simulink model "CCModel_62"  (R2024a)
settings: Solver=ode3  StartTime=0.0  StopTime=100  FixedStep=0.001  RelTol=1e-3  EnableMultiTasking=on
undefined symbols (not defined in the file or in its folder): DiscIntNeverNeededParam, Hecate_desVel1, Hecate_desVel2, Hecate_desVel3, Hecate_horShift, Hecate_period, Hecate_slope, Hecate_Transition1, Hecate_Transition2, Hecate_verShift, i, PME_qb, qb_map, RPM_qb, V
libraries: simulink x46
(part 11 of 11)

== system CCModel_62/Cruise Control/Version 6.1/Switches/Sigmoid_brake ==
  Change_time : Inport
  Old brake : Inport  Port=2
  New brake : Inport  Port=3
  Add : Sum
  Add1 : Sum
  Add2 : Sum
  Clock : Clock
  Constant : Constant
  Constant1 : Constant
  Constant2 : Constant
  Divide : Product  Inputs=/*
  Divide1 : Product  Inputs=**
  Divide2 : Product  Inputs=/*
  Divide3 : Product  Inputs=**
  Gain : Gain  Gain=1000
  Gain1 : Gain  Gain=0.001
  K : Constant
  Power{,1..3} (4 alike) : Math  Operator=pow
  Reciprocal : Product  Inputs=/
  Reciprocal1 : Product  Inputs=/
  Round : Rounding  Operator=round
  Scope : Scope  NumInputPorts=3
  Subtract : Sum  Inputs=-+
  Sum : Sum  Inputs=|-+
  brake_out : Outport
  wires:
  Power1/1 -> Scope/3, Add/1
  Add/1 -> Power/1
  Clock/1 -> Sum/2
  Constant/1 -> Add/2
  Sum/1 -> Gain/1  "Elapsed Time"
  Reciprocal/1 -> Power/2
  Power/1 -> Divide/1
  Divide/1 -> Divide1/1  "Sigmoid Function"
  Add1/1 -> Power2/1
  Power3/1 -> Add1/1
  K/1 -> Scope/2, Reciprocal/1, Power1/2, Reciprocal1/1, Power3/2
  Reciprocal1/1 -> Power2/2
  Power2/1 -> Divide2/1
  Constant1/1 -> Add1/2
  Change_time/1 -> Sum/1
  Constant2/1 -> Subtract/2
  Divide2/1 -> Subtract/1  "Sigmoid Function"
  Divide1/1 -> Add2/1
  Add2/1 -> brake_out/1
  New brake/1 -> Divide1/2
  Old brake/1 -> Divide3/2
  Subtract/1 -> Divide3/1
  Divide3/1 -> Add2/2
  Gain1/1 -> Power1/1, Divide/2, Scope/1, Divide2/2, Power3/1
  Gain/1 -> Round/1
  Round/1 -> Gain1/1

== system CCModel_62/Cruise Control/Version 6.1/Switches/Sigmoid_throttle ==
  Change_time : Inport
  Old thr : Inport  Port=2
  New thr : Inport  Port=3
  Add : Sum
  Add1 : Sum
  Add2 : Sum
  Clock : Clock
  Constant : Constant
  Constant1 : Constant
  Constant2 : Constant
  Divide : Product  Inputs=/*
  Divide1 : Product  Inputs=**
  Divide2 : Product  Inputs=/*
  Divide3 : Product  Inputs=**
  Gain : Gain  Gain=1000
  Gain1 : Gain  Gain=0.001
  K : Constant  Value=1.5
  Power{,1..3} (4 alike) : Math  Operator=pow
  Reciprocal : Product  Inputs=/
  Reciprocal1 : Product  Inputs=/
  Round : Rounding  Operator=round
  Scope : Scope  NumInputPorts=3
  Subtract : Sum  Inputs=-+
  Sum : Sum  Inputs=|-+
  throttle_out : Outport
  wires:
  Power1/1 -> Scope/3, Add/1
  Add/1 -> Power/1
  Clock/1 -> Sum/2
  Constant/1 -> Add/2
  Sum/1 -> Gain/1  "Elapsed Time"
  Reciprocal/1 -> Power/2
  Power/1 -> Divide/1
  Divide/1 -> Divide1/1  "Sigmoid Function"
  Add1/1 -> Power2/1
  Power3/1 -> Add1/1
  K/1 -> Scope/2, Reciprocal/1, Power1/2, Reciprocal1/1, Power3/2
  Reciprocal1/1 -> Power2/2
  Power2/1 -> Divide2/1
  Constant1/1 -> Add1/2
  Change_time/1 -> Sum/1
  Constant2/1 -> Subtract/2
  Divide2/1 -> Subtract/1  "Sigmoid Function"
  Divide1/1 -> Add2/1
  Add2/1 -> throttle_out/1
  New thr/1 -> Divide1/2
  Old thr/1 -> Divide3/2
  Subtract/1 -> Divide3/1
  Divide3/1 -> Add2/2
  Gain1/1 -> Power1/1, Divide/2, Scope/1, Divide2/2, Power3/1
  Gain/1 -> Round/1
  Round/1 -> Gain1/1

== system CCModel_62/Cruise Control/Version 6.2/Switches/Sigmoid_brake ==
  Change_time : Inport
  Old brake : Inport  Port=2
  New brake : Inport  Port=3
  Add : Sum
  Add1 : Sum
  Add2 : Sum
  Clock : Clock
  Constant : Constant
  Constant1 : Constant
  Constant2 : Constant
  Divide : Product  Inputs=/*
  Divide1 : Product  Inputs=**
  Divide2 : Product  Inputs=/*
  Divide3 : Product  Inputs=**
  Gain : Gain  Gain=1000
  Gain1 : Gain  Gain=0.001
  K : Constant  Value=1.5
  Power{,1..3} (4 alike) : Math  Operator=pow
  Reciprocal : Product  Inputs=/
  Reciprocal1 : Product  Inputs=/
  Round : Rounding  Operator=round
  Scope : Scope  NumInputPorts=3
  Subtract : Sum  Inputs=-+
  Sum : Sum  Inputs=|-+
  brake_out : Outport
  wires:
  Power1/1 -> Scope/3, Add/1
  Add/1 -> Power/1
  Clock/1 -> Sum/2
  Constant/1 -> Add/2
  Sum/1 -> Gain/1  "Elapsed Time"
  Reciprocal/1 -> Power/2
  Power/1 -> Divide/1
  Divide/1 -> Divide1/1  "Sigmoid Function"
  Add1/1 -> Power2/1
  Power3/1 -> Add1/1
  K/1 -> Scope/2, Reciprocal/1, Power1/2, Reciprocal1/1, Power3/2
  Reciprocal1/1 -> Power2/2
  Power2/1 -> Divide2/1
  Constant1/1 -> Add1/2
  Change_time/1 -> Sum/1
  Constant2/1 -> Subtract/2
  Divide2/1 -> Subtract/1  "Sigmoid Function"
  Divide1/1 -> Add2/1
  Add2/1 -> brake_out/1
  New brake/1 -> Divide1/2
  Old brake/1 -> Divide3/2
  Subtract/1 -> Divide3/1
  Divide3/1 -> Add2/2
  Gain1/1 -> Power1/1, Divide/2, Scope/1, Divide2/2, Power3/1
  Gain/1 -> Round/1
  Round/1 -> Gain1/1

== system CCModel_62/Cruise Control/Version 6.2/Switches/Sigmoid_throttle ==
  Change_time : Inport
  Old thr : Inport  Port=2
  New thr : Inport  Port=3
  Add : Sum
  Add1 : Sum
  Add2 : Sum
  Clock : Clock
  Constant : Constant
  Constant1 : Constant
  Constant2 : Constant
  Divide : Product  Inputs=/*
  Divide1 : Product  Inputs=**
  Divide2 : Product  Inputs=/*
  Divide3 : Product  Inputs=**
  Gain : Gain  Gain=1000
  Gain1 : Gain  Gain=0.001
  K : Constant  Value=1.5
  Power{,1..3} (4 alike) : Math  Operator=pow
  Reciprocal : Product  Inputs=/
  Reciprocal1 : Product  Inputs=/
  Round : Rounding  Operator=round
  Scope : Scope  NumInputPorts=3
  Subtract : Sum  Inputs=-+
  Sum : Sum  Inputs=|-+
  throttle_out : Outport
  wires:
  Power1/1 -> Scope/3, Add/1
  Add/1 -> Power/1
  Clock/1 -> Sum/2
  Constant/1 -> Add/2
  Sum/1 -> Gain/1  "Elapsed Time"
  Reciprocal/1 -> Power/2
  Power/1 -> Divide/1
  Divide/1 -> Divide1/1  "Sigmoid Function"
  Add1/1 -> Power2/1
  Power3/1 -> Add1/1
  K/1 -> Scope/2, Reciprocal/1, Power1/2, Reciprocal1/1, Power3/2
  Reciprocal1/1 -> Power2/2
  Power2/1 -> Divide2/1
  Constant1/1 -> Add1/2
  Change_time/1 -> Sum/1
  Constant2/1 -> Subtract/2
  Divide2/1 -> Subtract/1  "Sigmoid Function"
  Divide1/1 -> Add2/1
  Add2/1 -> throttle_out/1
  New thr/1 -> Divide1/2
  Old thr/1 -> Divide3/2
  Subtract/1 -> Divide3/1
  Divide3/1 -> Add2/2
  Gain1/1 -> Power1/1, Divide/2, Scope/1, Divide2/2, Power3/1
  Gain/1 -> Round/1
  Round/1 -> Gain1/1

== system CCModel_62/Cruise Control/Version 7.3/Detect Change/Change_Desired_Speed ==

== system CCModel_62/Cruise Control/Version 7.3/Detect Change/Driver Control ==

== system CCModel_62/Cruise Control/Version 7.3/Detect Change/Error_Equal_Zero ==

== system CCModel_62/Cruise Control/Version 7.3/PID Controller/Throttle Adjustment ==

== system CCModel_62/Powertrain/EM0/efficiency/divider ==
  In1 : Inport
  In2 : Inport  Port=2
  Fcn : Fcn  Expr="u(1) /  (u(2)+(u(2)==0) ) *(u(2)!=0)"
  Mux : Mux  Inputs=2
  Out1 : Outport
  wires:
  In2/1 -> Mux/2
  Fcn/1 -> Out1/1
  In1/1 -> Mux/1
  Mux/1 -> Fcn/1

== system CCModel_62/Powertrain/EM0/efficiency/divider1 ==
  In1 : Inport
  In2 : Inport  Port=2
  Fcn : Fcn  Expr="u(1) /  (u(2)+(u(2)==0) ) *(u(2)!=0)"
  Mux : Mux  Inputs=2
  Out1 : Outport
  wires:
  In2/1 -> Mux/2
  Fcn/1 -> Out1/1
  In1/1 -> Mux/1
  Mux/1 -> Fcn/1

== system CCModel_62/Powertrain/EM1/efficiency/divider ==
  In1 : Inport
  In2 : Inport  Port=2
  Fcn : Fcn  Expr="u(1) /  (u(2)+(u(2)==0) ) *(u(2)!=0)"
  Mux : Mux  Inputs=2
  Out1 : Outport
  wires:
  In2/1 -> Mux/2
  Fcn/1 -> Out1/1
  In1/1 -> Mux/1
  Mux/1 -> Fcn/1

== system CCModel_62/Powertrain/EM1/efficiency/divider1 ==
  In1 : Inport
  In2 : Inport  Port=2
  Fcn : Fcn  Expr="u(1) /  (u(2)+(u(2)==0) ) *(u(2)!=0)"
  Mux : Mux  Inputs=2
  Out1 : Outport
  wires:
  In2/1 -> Mux/2
  Fcn/1 -> Out1/1
  In1/1 -> Mux/1
  Mux/1 -> Fcn/1

== system CCModel_62/Powertrain/EM2/efficiency/divider ==
  In1 : Inport
  In2 : Inport  Port=2
  Fcn : Fcn  Expr="u(1) /  (u(2)+(u(2)==0) ) *(u(2)!=0)"
  Mux : Mux  Inputs=2
  Out1 : Outport
  wires:
  In2/1 -> Mux/2
  Fcn/1 -> Out1/1
  In1/1 -> Mux/1
  Mux/1 -> Fcn/1

== system CCModel_62/Powertrain/EM2/efficiency/divider1 ==
  In1 : Inport
  In2 : Inport  Port=2
  Fcn : Fcn  Expr="u(1) /  (u(2)+(u(2)==0) ) *(u(2)!=0)"
  Mux : Mux  Inputs=2
  Out1 : Outport
  wires:
  In2/1 -> Mux/2
  Fcn/1 -> Out1/1
  In1/1 -> Mux/1
  Mux/1 -> Fcn/1

== system CCModel_62/Powertrain/EM3/efficiency/divider ==
  In1 : Inport
  In2 : Inport  Port=2
  Fcn : Fcn  Expr="u(1) /  (u(2)+(u(2)==0) ) *(u(2)!=0)"
  Mux : Mux  Inputs=2
  Out1 : Outport
  wires:
  In2/1 -> Mux/2
  Fcn/1 -> Out1/1
  In1/1 -> Mux/1
  Mux/1 -> Fcn/1

== system CCModel_62/Powertrain/EM3/efficiency/divider1 ==
  In1 : Inport
  In2 : Inport  Port=2
  Fcn : Fcn  Expr="u(1) /  (u(2)+(u(2)==0) ) *(u(2)!=0)"
  Mux : Mux  Inputs=2
  Out1 : Outport
  wires:
  In2/1 -> Mux/2
  Fcn/1 -> Out1/1
  In1/1 -> Mux/1
  Mux/1 -> Fcn/1

== system CCModel_62/Powertrain/EM4Front/efficiency/divider ==
  In1 : Inport
  In2 : Inport  Port=2
  Fcn : Fcn  Expr="u(1) /  (u(2)+(u(2)==0) ) *(u(2)!=0)"
  Mux : Mux  Inputs=2
  Out1 : Outport
  wires:
  In2/1 -> Mux/2
  Fcn/1 -> Out1/1
  In1/1 -> Mux/1
  Mux/1 -> Fcn/1

== system CCModel_62/Powertrain/EM4Front/efficiency/divider1 ==
  In1 : Inport
  In2 : Inport  Port=2
  Fcn : Fcn  Expr="u(1) /  (u(2)+(u(2)==0) ) *(u(2)!=0)"
  Mux : Mux  Inputs=2
  Out1 : Outport
  wires:
  In2/1 -> Mux/2
  Fcn/1 -> Out1/1
  In1/1 -> Mux/1
  Mux/1 -> Fcn/1

== system CCModel_62/Powertrain/EM4Rear/efficiency/divider ==
  In1 : Inport
  In2 : Inport  Port=2
  Fcn : Fcn  Expr="u(1) /  (u(2)+(u(2)==0) ) *(u(2)!=0)"
  Mux : Mux  Inputs=2
  Out1 : Outport
  wires:
  In2/1 -> Mux/2
  Fcn/1 -> Out1/1
  In1/1 -> Mux/1
  Mux/1 -> Fcn/1

== system CCModel_62/Powertrain/EM4Rear/efficiency/divider1 ==
  In1 : Inport
  In2 : Inport  Port=2
  Fcn : Fcn  Expr="u(1) /  (u(2)+(u(2)==0) ) *(u(2)!=0)"
  Mux : Mux  Inputs=2
  Out1 : Outport
  wires:
  In2/1 -> Mux/2
  Fcn/1 -> Out1/1
  In1/1 -> Mux/1
  Mux/1 -> Fcn/1

== system CCModel_62/Powertrain/EMR/efficiency/divider ==
  In1 : Inport
  In2 : Inport  Port=2
  Fcn : Fcn  Expr="u(1) /  (u(2)+(u(2)==0) ) *(u(2)!=0)"
  Mux : Mux  Inputs=2
  Out1 : Outport
  wires:
  In2/1 -> Mux/2
  Fcn/1 -> Out1/1
  In1/1 -> Mux/1
  Mux/1 -> Fcn/1

== system CCModel_62/Powertrain/EMR/efficiency/divider1 ==
  In1 : Inport
  In2 : Inport  Port=2
  Fcn : Fcn  Expr="u(1) /  (u(2)+(u(2)==0) ) *(u(2)!=0)"
  Mux : Mux  Inputs=2
  Out1 : Outport
  wires:
  In2/1 -> Mux/2
  Fcn/1 -> Out1/1
  In1/1 -> Mux/1
  Mux/1 -> Fcn/1

== system CCModel_62/Powertrain/EMS/efficiency/divider ==
  In1 : Inport
  In2 : Inport  Port=2
  Fcn : Fcn  Expr="u(1) /  (u(2)+(u(2)==0) ) *(u(2)!=0)"
  Mux : Mux  Inputs=2
  Out1 : Outport
  wires:
  In2/1 -> Mux/2
  Fcn/1 -> Out1/1
  In1/1 -> Mux/1
  Mux/1 -> Fcn/1

== system CCModel_62/Powertrain/EMS/efficiency/divider1 ==
  In1 : Inport
  In2 : Inport  Port=2
  Fcn : Fcn  Expr="u(1) /  (u(2)+(u(2)==0) ) *(u(2)!=0)"
  Mux : Mux  Inputs=2
  Out1 : Outport
  wires:
  In2/1 -> Mux/2
  Fcn/1 -> Out1/1
  In1/1 -> Mux/1
  Mux/1 -> Fcn/1

== system CCModel_62/Powertrain/EV/Motor Efficiency/  ==
  In1 : Inport
  In2 : Inport  Port=2
  Fcn : Fcn  Expr=u[1]/(u[2]+(u[2]==0))*(u[2]!=0)
  Mux : Mux  Inputs=2
  Out1 : Outport  VectorParamsAs1DForOutWhenUnconnected=off
  wires:
  In1/1 -> Mux/1
  In2/1 -> Mux/2
  Mux/1 -> Fcn/1
  Fcn/1 -> Out1/1

== system CCModel_62/Powertrain/GEN/efficiency/divider ==
  In1 : Inport
  In2 : Inport  Port=2
  Fcn : Fcn  Expr="u(1) /  (u(2)+(u(2)==0) ) *(u(2)!=0)"
  Mux : Mux  Inputs=2
  Out1 : Outport
  wires:
  In2/1 -> Mux/2
  Fcn/1 -> Out1/1
  In1/1 -> Mux/1
  Mux/1 -> Fcn/1

== system CCModel_62/Powertrain/GEN/efficiency/divider1 ==
  In1 : Inport
  In2 : Inport  Port=2
  Fcn : Fcn  Expr="u(1) /  (u(2)+(u(2)==0) ) *(u(2)!=0)"
  Mux : Mux  Inputs=2
  Out1 : Outport
  wires:
  In2/1 -> Mux/2
  Fcn/1 -> Out1/1
  In1/1 -> Mux/1
  Mux/1 -> Fcn/1

== system CCModel_62/Powertrain/MOT/efficiency/divider ==
  In1 : Inport
  In2 : Inport  Port=2
  Fcn : Fcn  Expr="u(1) /  (u(2)+(u(2)==0) ) *(u(2)!=0)"
  Mux : Mux  Inputs=2
  Out1 : Outport
  wires:
  In2/1 -> Mux/2
  Fcn/1 -> Out1/1
  In1/1 -> Mux/1
  Mux/1 -> Fcn/1

== system CCModel_62/Powertrain/MOT/efficiency/divider1 ==
  In1 : Inport
  In2 : Inport  Port=2
  Fcn : Fcn  Expr="u(1) /  (u(2)+(u(2)==0) ) *(u(2)!=0)"
  Mux : Mux  Inputs=2
  Out1 : Outport
  wires:
  In2/1 -> Mux/2
  Fcn/1 -> Out1/1
  In1/1 -> Mux/1
  Mux/1 -> Fcn/1

== stateflow chart CCModel_62/Requirements Table ==
  (default) -> (junction 1073742629)
  (junction 1073742629) -> (junction 1073742630) : {
      | % SF_REQ_REV_07
      | }
  (junction 1073742630) -> (junction 1073742632) : {
      | % ExcEvals:
      | % PriEvals:
      | }
  (junction 1073742632) -> (junction 1073742634) : {
      | % HEADER_ASSIGNMENTS
      |
      | }
  (junction 1073742634) -> (junction 1073742636) : {
      | % START_A_4
      | }
  (junction 1073742636) -> (junction 1073742638) : {
      | }
  (junction 1073742638) -> (junction 1073742640)
  (junction 1073742640) -> (junction 1073742642) : {
      | }
  (junction 1073742642) -> (junction 1073742644) : {
      | % END_A_4
      | }
  (junction 1073742644) -> (junction 1073742646) : {
      | % START_R_1
      | }
  (junction 1073742646) -> (junction 1073742648) : {
      | }
  (junction 1073742648) -> (junction 1073742650)
  (junction 1073742650) -> (junction 1073742652) [order 1] : [duration((((throttle) < (1))) && (((brake) < (1)))) >= 0.5]
  (junction 1073742650) -> (junction 1073742658) [order 2]
  (junction 1073742652) -> (junction 1073742654) : {
      | reqtable_postcondition((((long_acc) >= (-3.5) && (long_acc) <= (5))), 'R:1');
      |
      |
      | }
  (junction 1073742654) -> (junction 1073742656) : {
      | }
  (junction 1073742656) -> (junction 1073742658)
  (junction 1073742658) -> (junction 1073742660)
  (junction 1073742660) -> (junction 1073742662) : {
      | % END_R_1
      | }
  (junction 1073742662) -> (junction 1073742664) : {
      | % START_R_7
      | }
  (junction 1073742664) -> (junction 1073742666) : {
      | }
  (junction 1073742666) -> (junction 1073742668)
  (junction 1073742668) -> (junction 1073742670) [order 1] : [duration((((throttle) < (1))) && (((brake) < (1)))) >= 0.5]
  (junction 1073742668) -> (junction 1073742676) [order 2]
  (junction 1073742670) -> (junction 1073742672) : {
      | reqtable_postcondition((abs((jerk)) <10 ), 'R:2');
      |
      |
      | }
  (junction 1073742672) -> (junction 1073742674) : {
      | }
  (junction 1073742674) -> (junction 1073742676)
  (junction 1073742676) -> (junction 1073742678)
  (junction 1073742678) -> (junction 1073742680) : {
      | % END_R_7
      | }
  (junction 1073742680) -> (junction 1073742682) : {
      | % START_R_10
      | }
  (junction 1073742682) -> (junction 1073742684) : {
      | }
  (junction 1073742684) -> (junction 1073742686)
  (junction 1073742686) -> (junction 1073742688) [order 1] : [duration((((throttle) < (1))) && (((brake) < (1)))) >= 0.5]
  (junction 1073742686) -> (junction 1073742694) [order 2]
  (junction 1073742688) -> (junction 1073742690) : {
      | reqtable_postcondition((abs((pitch_acc)) <3), 'R:3');
      |
      |
      | }
  (junction 1073742690) -> (junction 1073742692) : {
      | }
  (junction 1073742692) -> (junction 1073742694)
  (junction 1073742694) -> (junction 1073742696)
  (junction 1073742696) -> (junction 1073742698) : {
      | % END_R_10
      | }
  (junction 1073742698) -> (junction 1073742700) : {
      | % START_R_13
      | }
  (junction 1073742700) -> (junction 1073742702) : {
      | }
  (junction 1073742702) -> (junction 1073742704)
  (junction 1073742704) -> (junction 1073742706) [order 1] : [duration((((throttle) < (1))) && (((brake) < (1))) && (~changeTrigger)) >= 30]
  (junction 1073742704) -> (junction 1073742712) [order 2]
  (junction 1073742706) -> (junction 1073742708) : {
      | reqtable_postcondition((abs(des_vel - long_vel) < 3), 'R:4');
      |
      |
      | }
  (junction 1073742708) -> (junction 1073742710) : {
      | }
  (junction 1073742710) -> (junction 1073742712)
  (junction 1073742712) -> (junction 1073742714)
  (junction 1073742714) -> (junction 1073742716) : {
      | % END_R_13
      | }
  (junction 1073742716) -> (junction 1073742718) : {
      | % START_R_16
      | }
  (junction 1073742718) -> (junction 1073742720) : {
      | }
  (junction 1073742720) -> (junction 1073742722)
  (junction 1073742722) -> (junction 1073742724) [order 1] : [(((throttle) < (100000000))) && (((brake) < (100000000)))]
  (junction 1073742722) -> (junction 1073742730) [order 2]
  (junction 1073742724) -> (junction 1073742726) : {
      | reqtable_postcondition((((long_acc) < (100000000))) && (((jerk) < (100000000))) && (((pitch_acc) < (100000000))) && (des_vel < 100000000 && long_vel < 100000000 ), 'R:5');
      |
      |
      | }
  (junction 1073742726) -> (junction 1073742728) : {
      | }
  (junction 1073742728) -> (junction 1073742730)
  (junction 1073742730) -> (junction 1073742732)
  (junction 1073742732) -> (junction 1073742734) : {
      | % END_R_16
      | }
  data: brake input; throttle input; long_acc input; jerk input; des_vel input; long_vel input; pitch_acc input; changeTrigger input

== stateflow chart CCModel_62/Test Sequence1 ==
  state TS1
    state step_1
      throttle_const = 0;
      brake_const=0;
      desired_velocity = Hecate_desVel1;
      grade = 0;
    state step_2
      desired_velocity = Hecate_desVel2;
    (default) -> TS1.step_1
    TS1.step_1 -> TS1.step_2 : [
        | et >= Hecate_Transition1
        | ]
  state TS2
    state step_1
      throttle_const = 100;
      brake_const = 0;
      desired_velocity = Hecate_desVel1;
      grade = 0;
    state step_2
      throttle_const = 70 - 0.1*et(msec);
    state step_3
      %do nothing
    state step_4
      desired_velocity = Hecate_desVel2;
    (default) -> TS2.step_1
    TS2.step_1 -> TS2.step_2 : [
        | velocity >= 50
        | ]
    TS2.step_2 -> TS2.step_3 : [
        | throttle_const <= 0
        | ]
    TS2.step_3 -> TS2.step_4 : [
        | et>=Hecate_Transition1
        | ]
  state TS3
    state step_1
      steer_angle = 0;
      throttle_const = 100;
      brake_const = 0;
      desired_velocity = Hecate_desVel1;
      grade = 0;
    state step_2
      throttle_const = 70 - 0.1*et(msec);
    state step_3
      %do nothing
    state step_4
      desired_velocity = Hecate_desVel2;
    state step_5
      desired_velocity = Hecate_desVel3;
    (default) -> TS3.step_1
    TS3.step_1 -> TS3.step_2 : [
        | velocity >= 50
        | ]
    TS3.step_2 -> TS3.step_3 : [
        | throttle_const <= 0
        | ]
    TS3.step_3 -> TS3.step_4 : [
        | et>=Hecate_Transition1
        | ]
    TS3.step_4 -> TS3.step_5 : [
        | et>=Hecate_Transition2
        | ]
  state TS4
    state step_1
      throttle_const = 100;
      brake_const = 0;
      desired_velocity = Hecate_desVel1;
      grade = Hecate_slope;
    state step_2
      throttle_const = 70 - 0.1*et(msec);
    state step_3
      %do nothing
    state step_4
      desired_velocity = Hecate_desVel2;
    (default) -> TS4.step_1
    TS4.step_1 -> TS4.step_2 : [
        | velocity >= 50
        | ]
    TS4.step_2 -> TS4.step_3 : [
        | throttle_const <= 0
        | ]
    TS4.step_3 -> TS4.step_4 : [
        | et>=Hecate_Transition1
        | ]
  state TS5
    state step_1
      steer_angle = 0;
      throttle_const = 100;
      brake_const = 0;
      desired_velocity = Hecate_desVel1;
      grade = Hecate_slope;
    state step_2
      throttle_const = 70 - 0.1*et(msec);
    state step_3
      %do nothing
    state step_4
      desired_velocity = Hecate_desVel2;
    state step_5
      desired_velocity = Hecate_desVel3;
    (default) -> TS5.step_1
    TS5.step_1 -> TS5.step_2 : [
        | velocity >= 50
        | ]
    TS5.step_2 -> TS5.step_3 : [
        | throttle_const <= 0
        | ]
    TS5.step_3 -> TS5.step_4 : [
        | et>=Hecate_Transition1
        | ]
    TS5.step_4 -> TS5.step_5 : [
        | et>=Hecate_Transition2
        | ]
  state TS6
    state Start_Up
      steer_angle = 0;
      throttle_const = 100;
      brake_const = 0;
      desired_velocity = Hecate_desVel1;
      grade = Hecate_slope*sin(pi*t/Hecate_period + Hecate_horShift) + Hecate_verShift;
    state Release_Throttle
      throttle_const = 70 - 0.1*et(msec);
      grade = Hecate_slope*sin(pi*t/Hecate_period + Hecate_horShift) + Hecate_verShift;
    state Initial_Step
      desired_velocity = Hecate_desVel1;
      grade = Hecate_slope*sin(pi*t/Hecate_period + Hecate_horShift) + Hecate_verShift;
    state Intermediary_Step
      desired_velocity = Hecate_desVel2;
      grade = Hecate_slope*sin(pi*t/Hecate_period + Hecate_horShift) + Hecate_verShift;
    state Final_Step
      desired_velocity = Hecate_desVel3;
      grade = Hecate_slope*sin(pi*t/Hecate_period + Hecate_horShift) + Hecate_verShift;
    (default) -> Start_Up
    Start_Up -> Release_Throttle : [
        | velocity >= 50
        | ]
    Release_Throttle -> Initial_Step : [
        | throttle_const <= 0
        | ]
    Initial_Step -> Intermediary_Step : [
        | et>=Hecate_Transition1
        | ]
    Intermediary_Step -> Final_Step : [
        | et>=Hecate_Transition2
        | ]
  state Scenario_1
    state step_1
    state step_2
    (default) -> Scenario_1.step_1
    Scenario_1.step_1 -> Scenario_1.step_2
  (default) -> TS1 [order 1] : [Active_Scenario_Index == 1]
  (default) -> TS2 [order 2] : [Active_Scenario_Index == 2]
  (default) -> TS3 [order 3] : [Active_Scenario_Index == 3]
  (default) -> TS4 [order 4] : [Active_Scenario_Index == 4]
  (default) -> TS5 [order 5] : [Active_Scenario_Index == 5]
  (default) -> TS6 [order 6] : [Active_Scenario_Index == 6]
  (default) -> Scenario_1 [order 7] : {assert(Active_Scenario_Index == 7,'The value of Scenario Parameter ''Active_Scenario_Index'' is not valid. Use the index of the scenario to specify it.')}
  data: steer_angle output; throttle_const output; brake_const output; Active_Scenario_Index parameter =4; Hecate_desVel2 parameter; Hecate_desVel1 parameter; desired_velocity output; Hecate_desVel3 parameter; Hecate_Transition1 parameter; Hecate_Transition2 parameter; velocity input; grade output; Hecate_slope parameter; Hecate_horShift parameter; Hecate_verShift parameter; Hecate_period parameter

== stateflow chart CCModel_62/FitnessConverter_Hecate ==
  state Requirement_1 [parallel]
    settings: executionOrder=1
    state Default
      rob1 = Inf;
    state Wait
      rob1 = Inf;
    state Verify
      rob1 = min( 5-(long_acc),(long_acc-( -3.5)));
    (default) -> (junction 14)
    (junction 14) -> Requirement_1.Wait [order 2]
    (junction 14) -> Requirement_1.Default [order 1] : [~((throttle<1) && (brake<1))]
    Requirement_1.Default -> Requirement_1.Wait : [(throttle<1) && (brake<1)]
    Requirement_1.Wait -> Requirement_1.Default [order 1] : [~((throttle<1) && (brake<1))]
    Requirement_1.Verify -> Requirement_1.Default : [~((throttle<1) && (brake<1))]
    Requirement_1.Wait -> Requirement_1.Verify [order 2] : [et >= 0.5]
  state Requirement_2 [parallel]
    settings: executionOrder=2
    state Default
      rob2 = Inf;
    state Wait
      rob2 = Inf;
    state Verify
      rob2 = 10-((abs(jerk)));
    (default) -> (junction 26)
    (junction 26) -> Requirement_2.Wait [order 2]
    (junction 26) -> Requirement_2.Default [order 1] : [~((throttle<1) && (brake<1))]
    Requirement_2.Default -> Requirement_2.Wait : [(throttle<1) && (brake<1)]
    Requirement_2.Wait -> Requirement_2.Default [order 1] : [~((throttle<1) && (brake<1))]
    Requirement_2.Verify -> Requirement_2.Default : [~((throttle<1) && (brake<1))]
    Requirement_2.Wait -> Requirement_2.Verify [order 2] : [et >= 0.5]
  state Requirement_3 [parallel]
    settings: executionOrder=3
    state Default
      rob3 = Inf;
    state Wait
      rob3 = Inf;
    state Verify
      rob3 = 3-((abs(pitch_acc)));
    (default) -> (junction 38)
    (junction 38) -> Requirement_3.Wait [order 2]
    (junction 38) -> Requirement_3.Default [order 1] : [~((throttle<1) && (brake<1))]
    Requirement_3.Default -> Requirement_3.Wait : [(throttle<1) && (brake<1)]
    Requirement_3.Wait -> Requirement_3.Default [order 1] : [~((throttle<1) && (brake<1))]
    Requirement_3.Verify -> Requirement_3.Default : [~((throttle<1) && (brake<1))]
    Requirement_3.Wait -> Requirement_3.Verify [order 2] : [et >= 0.5]
  state Requirement_4 [parallel]
    settings: executionOrder=4
    state Default
      rob4 = Inf;
    state Wait
      rob4 = Inf;
    state Verify
      rob4 = 3-((abs(des_vel-long_vel)));
    (default) -> (junction 50)
    (junction 50) -> Requirement_4.Wait [order 2]
    (junction 50) -> Requirement_4.Default [order 1] : [~((throttle<1) && (brake<1) && (~changeTrigger))]
    Requirement_4.Default -> Requirement_4.Wait : [(throttle<1) && (brake<1) && (~changeTrigger)]
    Requirement_4.Wait -> Requirement_4.Default [order 1] : [~((throttle<1) && (brake<1) && (~changeTrigger))]
    Requirement_4.Verify -> Requirement_4.Default : [~((throttle<1) && (brake<1) && (~changeTrigger))]
    Requirement_4.Wait -> Requirement_4.Verify [order 2] : [et >= 30]
  data: brake input; throttle input; long_acc input; jerk input; des_vel input; long_vel input; pitch_acc input; changeTrigger input; rob1 output double =Inf; rob2 output double =Inf; rob3 output double =Inf; rob4 output double =Inf

== stateflow chart CCModel_62/Test Assessment1 ==
  state Func
    state Driver_Active
      %Do nothing
      settings: description=Recent brake
    state Buffer
      %Wait
    state CC_Active
      %Nothing
      settings: description=Start
      state Wait_Period
        %Nothing
        settings: description=Recent change (start)
      state Time_Threshold
        verify(abs(desired_velocity-long_vel_lp) <= 3)
        settings: description=No recent change
      state Refresh
        %Nothing
      Func.CC_Active.Refresh -> (junction 350) : [
          | et >= 0.5
          | ]
      (default) -> Func.CC_Active.Wait_Period
      Func.CC_Active.Wait_Period -> (junction 344) [order 2] : [
          | hasChanged(desired_velocity)
          | ]
      (junction 348) -> Func.CC_Active.Wait_Period
      (junction 344) -> (junction 342)
      Func.CC_Active.Wait_Period -> Func.CC_Active.Time_Threshold [order 1] : [
          | et >= 29.5
          | ]
      Func.CC_Active.Time_Threshold -> Func.CC_Active.Refresh : [
          | hasChanged(desired_velocity)
          | ]
      (junction 342) -> Func.CC_Active.Refresh
      (junction 350) -> (junction 348)
    Func.CC_Active -> (junction 338) : [
        | brake >= 1 || throttle >= 1
        | ]
    (default) -> Func.Driver_Active
    (junction 336) -> Func.Driver_Active
    Func.Driver_Active -> Func.Buffer : [
        | brake < 1 && throttle < 1
        | ]
    Func.Buffer -> Func.CC_Active : [
        | et >= 0.5
        | ]
    (junction 338) -> (junction 336)
  state DrivAndFunc
    state Driver_Active
      %Do nothing
      settings: description=Recent brake
    state Buffer
      %Wait
    state CC_Active
      verify(long_acc_lp <= 5)
      verify(long_acc_lp >= -3.5)
      verify(abs(pitch_acc_lp) <=3)
      verify(abs(long_jerk) <= 10)
      settings: description=Start
      state Wait_Period
        %Nothing
        settings: description=Recent change (start)
      state Time_Threshold
        verify(abs(desired_velocity-long_vel_lp) <= 3)
        settings: description=No recent change
      state Refresh
        %Nothing
      DrivAndFunc.CC_Active.Refresh -> (junction 260) : [
          | et >= 0.5
          | ]
      (default) -> DrivAndFunc.CC_Active.Wait_Period
      DrivAndFunc.CC_Active.Wait_Period -> (junction 254) [order 2] : [
          | hasChanged(desired_velocity)
          | ]
      (junction 258) -> DrivAndFunc.CC_Active.Wait_Period
      (junction 254) -> (junction 252)
      DrivAndFunc.CC_Active.Wait_Period -> DrivAndFunc.CC_Active.Time_Threshold [order 1] : [
          | et >= 29.5
          | ]
      DrivAndFunc.CC_Active.Time_Threshold -> DrivAndFunc.CC_Active.Refresh : [
          | hasChanged(desired_velocity)
          | ]
      (junction 252) -> DrivAndFunc.CC_Active.Refresh
      (junction 260) -> (junction 258)
    DrivAndFunc.CC_Active -> (junction 248) : [
        | brake >= 1 || throttle >= 1
        | ]
    (default) -> DrivAndFunc.Driver_Active
    (junction 246) -> DrivAndFunc.Driver_Active
    DrivAndFunc.Driver_Active -> DrivAndFunc.Buffer : [
        | brake < 1 && throttle < 1
        | ]
    DrivAndFunc.Buffer -> DrivAndFunc.CC_Active : [
        | et >= 0.5
        | ]
    (junction 248) -> (junction 246)
  (default) -> Func [order 1] : [Active_Scenario_Index == 1]
  (default) -> DrivAndFunc [order 2] : {assert(Active_Scenario_Index == 2,'The value of Scenario Parameter ''Active_Scenario_Index'' is not valid. Use the index of the scenario to specify it.')}
  data: long_jerk input; long_acc_lp input; long_vel_lp input; pitch_acc_lp input; Active_Scenario_Index parameter =1; brake input; throttle input; desired_velocity input

== stateflow chart CCModel_62/Requirements Table1 ==
  (default) -> (junction 1073742629)
  (junction 1073742629) -> (junction 1073742630) : {
      | % SF_REQ_REV_07
      | }
  (junction 1073742630) -> (junction 1073742632) : {
      | % ExcEvals:
      | % PriEvals:
      | }
  (junction 1073742632) -> (junction 1073742634) : {
      | % HEADER_ASSIGNMENTS
      |
      | }
  (junction 1073742634) -> (junction 1073742636) : {
      | % START_A_4
      | }
  (junction 1073742636) -> (junction 1073742638) : {
      | }
  (junction 1073742638) -> (junction 1073742640)
  (junction 1073742640) -> (junction 1073742642) : {
      | }
  (junction 1073742642) -> (junction 1073742644) : {
      | % END_A_4
      | }
  (junction 1073742644) -> (junction 1073742646) : {
      | % START_R_1
      | }
  (junction 1073742646) -> (junction 1073742648) : {
      | }
  (junction 1073742648) -> (junction 1073742650)
  (junction 1073742650) -> (junction 1073742652) [order 1] : [duration((((throttle) < (1))) && (((brake) < (1)))) >= 0.7]
  (junction 1073742650) -> (junction 1073742658) [order 2]
  (junction 1073742652) -> (junction 1073742654) : {
      | reqtable_postcondition((((long_acc) >= (-3.5) && (long_acc) <= (5))), 'R:1');
      |
      |
      | }
  (junction 1073742654) -> (junction 1073742656) : {
      | }
  (junction 1073742656) -> (junction 1073742658)
  (junction 1073742658) -> (junction 1073742660)
  (junction 1073742660) -> (junction 1073742662) : {
      | % END_R_1
      | }
  (junction 1073742662) -> (junction 1073742664) : {
      | % START_R_7
      | }
  (junction 1073742664) -> (junction 1073742666) : {
      | }
  (junction 1073742666) -> (junction 1073742668)
  (junction 1073742668) -> (junction 1073742670) [order 1] : [duration((((throttle) < (1))) && (((brake) < (1)))) >= 0.7]
  (junction 1073742668) -> (junction 1073742676) [order 2]
  (junction 1073742670) -> (junction 1073742672) : {
      | reqtable_postcondition((abs((jerk)) <10 ), 'R:2');
      |
      |
      | }
  (junction 1073742672) -> (junction 1073742674) : {
      | }
  (junction 1073742674) -> (junction 1073742676)
  (junction 1073742676) -> (junction 1073742678)
  (junction 1073742678) -> (junction 1073742680) : {
      | % END_R_7
      | }
  (junction 1073742680) -> (junction 1073742682) : {
      | % START_R_10
      | }
  (junction 1073742682) -> (junction 1073742684) : {
      | }
  (junction 1073742684) -> (junction 1073742686)
  (junction 1073742686) -> (junction 1073742688) [order 1] : [duration((((throttle) < (1))) && (((brake) < (1)))) >= 0.7]
  (junction 1073742686) -> (junction 1073742694) [order 2]
  (junction 1073742688) -> (junction 1073742690) : {
      | reqtable_postcondition((abs((pitch_acc)) <3), 'R:3');
      |
      |
      | }
  (junction 1073742690) -> (junction 1073742692) : {
      | }
  (junction 1073742692) -> (junction 1073742694)
  (junction 1073742694) -> (junction 1073742696)
  (junction 1073742696) -> (junction 1073742698) : {
      | % END_R_10
      | }
  (junction 1073742698) -> (junction 1073742700) : {
      | % START_R_13
      | }
  (junction 1073742700) -> (junction 1073742702) : {
      | }
  (junction 1073742702) -> (junction 1073742704)
  (junction 1073742704) -> (junction 1073742706) [order 1] : [duration((((throttle) < (1))) && (((brake) < (1))) && (~changeTrigger)) >= 30]
  (junction 1073742704) -> (junction 1073742712) [order 2]
  (junction 1073742706) -> (junction 1073742708) : {
      | reqtable_postcondition((abs(des_vel - long_vel) < 3), 'R:4');
      |
      |
      | }
  (junction 1073742708) -> (junction 1073742710) : {
      | }
  (junction 1073742710) -> (junction 1073742712)
  (junction 1073742712) -> (junction 1073742714)
  (junction 1073742714) -> (junction 1073742716) : {
      | % END_R_13
      | }
  (junction 1073742716) -> (junction 1073742718) : {
      | % START_R_16
      | }
  (junction 1073742718) -> (junction 1073742720) : {
      | }
  (junction 1073742720) -> (junction 1073742722)
  (junction 1073742722) -> (junction 1073742724) [order 1] : [(((throttle) < (100000000))) && (((brake) < (100000000)))]
  (junction 1073742722) -> (junction 1073742730) [order 2]
  (junction 1073742724) -> (junction 1073742726) : {
      | reqtable_postcondition((((long_acc) < (100000000))) && (((jerk) < (100000000))) && (((pitch_acc) < (100000000))) && (des_vel < 100000000 && long_vel < 100000000 ), 'R:5');
      |
      |
      | }
  (junction 1073742726) -> (junction 1073742728) : {
      | }
  (junction 1073742728) -> (junction 1073742730)
  (junction 1073742730) -> (junction 1073742732)
  (junction 1073742732) -> (junction 1073742734) : {
      | % END_R_16
      | }
  data: brake input; throttle input; long_acc input; jerk input; des_vel input; long_vel input; pitch_acc input; changeTrigger input

== stateflow chart CCModel_62/Requirements Table2 ==
  (default) -> (junction 1073742629)
  (junction 1073742629) -> (junction 1073742630) : {
      | % SF_REQ_REV_07
      | }
  (junction 1073742630) -> (junction 1073742632) : {
      | % ExcEvals:
      | % PriEvals:
      | }
  (junction 1073742632) -> (junction 1073742634) : {
      | % HEADER_ASSIGNMENTS
      |
      | }
  (junction 1073742634) -> (junction 1073742636) : {
      | % START_A_4
      | }
  (junction 1073742636) -> (junction 1073742638) : {
      | }
  (junction 1073742638) -> (junction 1073742640)
  (junction 1073742640) -> (junction 1073742642) : {
      | }
  (junction 1073742642) -> (junction 1073742644) : {
      | % END_A_4
      | }
  (junction 1073742644) -> (junction 1073742646) : {
      | % START_R_1
      | }
  (junction 1073742646) -> (junction 1073742648) : {
      | }
  (junction 1073742648) -> (junction 1073742650)
  (junction 1073742650) -> (junction 1073742652) [order 1] : [duration((((throttle) < (1))) && (((brake) < (1)))) >= 0.7]
  (junction 1073742650) -> (junction 1073742658) [order 2]
  (junction 1073742652) -> (junction 1073742654) : {
      | reqtable_postcondition((((long_acc) >= (-3.5) && (long_acc) <= (5))), 'R:1');
      |
      |
      | }
  (junction 1073742654) -> (junction 1073742656) : {
      | }
  (junction 1073742656) -> (junction 1073742658)
  (junction 1073742658) -> (junction 1073742660)
  (junction 1073742660) -> (junction 1073742662) : {
      | % END_R_1
      | }
  (junction 1073742662) -> (junction 1073742664) : {
      | % START_R_7
      | }
  (junction 1073742664) -> (junction 1073742666) : {
      | }
  (junction 1073742666) -> (junction 1073742668)
  (junction 1073742668) -> (junction 1073742670) [order 1] : [duration((((throttle) < (1))) && (((brake) < (1)))) >= 0.7]
  (junction 1073742668) -> (junction 1073742676) [order 2]
  (junction 1073742670) -> (junction 1073742672) : {
      | reqtable_postcondition((abs((jerk)) <10 ), 'R:2');
      |
      |
      | }
  (junction 1073742672) -> (junction 1073742674) : {
      | }
  (junction 1073742674) -> (junction 1073742676)
  (junction 1073742676) -> (junction 1073742678)
  (junction 1073742678) -> (junction 1073742680) : {
      | % END_R_7
      | }
  (junction 1073742680) -> (junction 1073742682) : {
      | % START_R_10
      | }
  (junction 1073742682) -> (junction 1073742684) : {
      | }
  (junction 1073742684) -> (junction 1073742686)
  (junction 1073742686) -> (junction 1073742688) [order 1] : [duration((((throttle) < (1))) && (((brake) < (1)))) >= 0.7]
  (junction 1073742686) -> (junction 1073742694) [order 2]
  (junction 1073742688) -> (junction 1073742690) : {
      | reqtable_postcondition((abs((pitch_acc)) <3), 'R:3');
      |
      |
      | }
  (junction 1073742690) -> (junction 1073742692) : {
      | }
  (junction 1073742692) -> (junction 1073742694)
  (junction 1073742694) -> (junction 1073742696)
  (junction 1073742696) -> (junction 1073742698) : {
      | % END_R_10
      | }
  (junction 1073742698) -> (junction 1073742700) : {
      | % START_R_13
      | }
  (junction 1073742700) -> (junction 1073742702) : {
      | }
  (junction 1073742702) -> (junction 1073742704)
  (junction 1073742704) -> (junction 1073742706) [order 1] : [duration((((throttle) < (1))) && (((brake) < (1))) && (~changeTrigger)) >= 30]
  (junction 1073742704) -> (junction 1073742712) [order 2]
  (junction 1073742706) -> (junction 1073742708) : {
      | reqtable_postcondition((abs(des_vel - long_vel) < 4), 'R:4');
      |
      |
      | }
  (junction 1073742708) -> (junction 1073742710) : {
      | }
  (junction 1073742710) -> (junction 1073742712)
  (junction 1073742712) -> (junction 1073742714)
  (junction 1073742714) -> (junction 1073742716) : {
      | % END_R_13
      | }
  (junction 1073742716) -> (junction 1073742718) : {
      | % START_R_16
      | }
  (junction 1073742718) -> (junction 1073742720) : {
      | }
  (junction 1073742720) -> (junction 1073742722)
  (junction 1073742722) -> (junction 1073742724) [order 1] : [(((throttle) < (100000000))) && (((brake) < (100000000)))]
  (junction 1073742722) -> (junction 1073742730) [order 2]
  (junction 1073742724) -> (junction 1073742726) : {
      | reqtable_postcondition((((long_acc) < (100000000))) && (((jerk) < (100000000))) && (((pitch_acc) < (100000000))) && (des_vel < 100000000 && long_vel < 100000000 ), 'R:5');
      |
      |
      | }
  (junction 1073742726) -> (junction 1073742728) : {
      | }
  (junction 1073742728) -> (junction 1073742730)
  (junction 1073742730) -> (junction 1073742732)
  (junction 1073742732) -> (junction 1073742734) : {
      | % END_R_16
      | }
  data: brake input; throttle input; long_acc input; jerk input; des_vel input; long_vel input; pitch_acc input; changeTrigger input

== stateflow chart CCModel_62/Requirements Table3 ==
  (default) -> (junction 1073742629)
  (junction 1073742629) -> (junction 1073742630) : {
      | % SF_REQ_REV_07
      | }
  (junction 1073742630) -> (junction 1073742632) : {
      | % ExcEvals:
      | % PriEvals:
      | }
  (junction 1073742632) -> (junction 1073742634) : {
      | % HEADER_ASSIGNMENTS
      |
      | }
  (junction 1073742634) -> (junction 1073742636) : {
      | % START_A_4
      | }
  (junction 1073742636) -> (junction 1073742638) : {
      | }
  (junction 1073742638) -> (junction 1073742640)
  (junction 1073742640) -> (junction 1073742642) : {
      | }
  (junction 1073742642) -> (junction 1073742644) : {
      | % END_A_4
      | }
  (junction 1073742644) -> (junction 1073742646) : {
      | % START_R_1
      | }
  (junction 1073742646) -> (junction 1073742648) : {
      | }
  (junction 1073742648) -> (junction 1073742650)
  (junction 1073742650) -> (junction 1073742652) [order 1] : [duration((((throttle) < (1))) && (((brake) < (1)))) >= 0.7]
  (junction 1073742650) -> (junction 1073742658) [order 2]
  (junction 1073742652) -> (junction 1073742654) : {
      | reqtable_postcondition((((long_acc) >= (-3.5) && (long_acc) <= (5))), 'R:1');
      |
      |
      | }
  (junction 1073742654) -> (junction 1073742656) : {
      | }
  (junction 1073742656) -> (junction 1073742658)
  (junction 1073742658) -> (junction 1073742660)
  (junction 1073742660) -> (junction 1073742662) : {
      | % END_R_1
      | }
  (junction 1073742662) -> (junction 1073742664) : {
      | % START_R_7
      | }
  (junction 1073742664) -> (junction 1073742666) : {
      | }
  (junction 1073742666) -> (junction 1073742668)
  (junction 1073742668) -> (junction 1073742670) [order 1] : [duration((((throttle) < (1))) && (((brake) < (1)))) >= 0.7]
  (junction 1073742668) -> (junction 1073742676) [order 2]
  (junction 1073742670) -> (junction 1073742672) : {
      | reqtable_postcondition((abs((jerk)) <10 ), 'R:2');
      |
      |
      | }
  (junction 1073742672) -> (junction 1073742674) : {
      | }
  (junction 1073742674) -> (junction 1073742676)
  (junction 1073742676) -> (junction 1073742678)
  (junction 1073742678) -> (junction 1073742680) : {
      | % END_R_7
      | }
  (junction 1073742680) -> (junction 1073742682) : {
      | % START_R_10
      | }
  (junction 1073742682) -> (junction 1073742684) : {
      | }
  (junction 1073742684) -> (junction 1073742686)
  (junction 1073742686) -> (junction 1073742688) [order 1] : [duration((((throttle) < (1))) && (((brake) < (1)))) >= 0.7]
  (junction 1073742686) -> (junction 1073742694) [order 2]
  (junction 1073742688) -> (junction 1073742690) : {
      | reqtable_postcondition((abs((pitch_acc)) <3), 'R:3');
      |
      |
      | }
  (junction 1073742690) -> (junction 1073742692) : {
      | }
  (junction 1073742692) -> (junction 1073742694)
  (junction 1073742694) -> (junction 1073742696)
  (junction 1073742696) -> (junction 1073742698) : {
      | % END_R_10
      | }
  (junction 1073742698) -> (junction 1073742700) : {
      | % START_R_13
      | }
  (junction 1073742700) -> (junction 1073742702) : {
      | }
  (junction 1073742702) -> (junction 1073742704)
  (junction 1073742704) -> (junction 1073742706) [order 1] : [duration((((throttle) < (1))) && (((brake) < (1))) && (~changeTrigger)) >= 30]
  (junction 1073742704) -> (junction 1073742712) [order 2]
  (junction 1073742706) -> (junction 1073742708) : {
      | reqtable_postcondition((abs(des_vel - long_vel) < 5), 'R:4');
      |
      |
      | }
  (junction 1073742708) -> (junction 1073742710) : {
      | }
  (junction 1073742710) -> (junction 1073742712)
  (junction 1073742712) -> (junction 1073742714)
  (junction 1073742714) -> (junction 1073742716) : {
      | % END_R_13
      | }
  (junction 1073742716) -> (junction 1073742718) : {
      | % START_R_16
      | }
  (junction 1073742718) -> (junction 1073742720) : {
      | }
  (junction 1073742720) -> (junction 1073742722)
  (junction 1073742722) -> (junction 1073742724) [order 1] : [(((throttle) < (100000000))) && (((brake) < (100000000)))]
  (junction 1073742722) -> (junction 1073742730) [order 2]
  (junction 1073742724) -> (junction 1073742726) : {
      | reqtable_postcondition((((long_acc) < (100000000))) && (((jerk) < (100000000))) && (((pitch_acc) < (100000000))) && (des_vel < 100000000 && long_vel < 100000000 ), 'R:5');
      |
      |
      | }
  (junction 1073742726) -> (junction 1073742728) : {
      | }
  (junction 1073742728) -> (junction 1073742730)
  (junction 1073742730) -> (junction 1073742732)
  (junction 1073742732) -> (junction 1073742734) : {
      | % END_R_16
      | }
  data: brake input; throttle input; long_acc input; jerk input; des_vel input; long_vel input; pitch_acc input; changeTrigger input
